simulink model "speedControlSystem"  (R2024b)
settings: Solver=FixedStepAuto  StartTime=0.0  StopTime=Tend  FixedStep=Tsim  RelTol=1e-3
values from neighbouring files (symbols this model uses):
  b = 4.28e-6    (= 4.28e-06)    [setup.m]    (also in test.m)
  encoder_noise_power = 0.5e-6*0    (= 0)    [test.m]
  J = 29.54e-6    (= 2.954e-05)    [test.m]
  speed_ref = 5e3    (= 5000)    [test.m]
  Tend = 10    [computing_speed.m]    (also in setup.m = 0.2; test.m = 0.2)
  Tsim = 1e-5    (= 1e-05)    [computing_speed.m]    (also in setup.m; test.m = 0.0001)
libraries: simulink x1
settings Model: Creator=mhmok  LastModifiedBy=mhmok

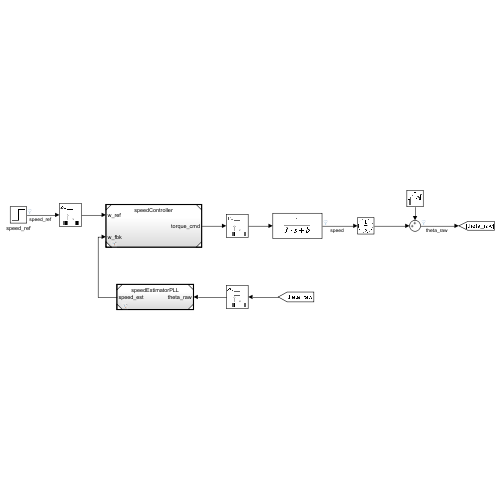
[thumbnail: Simulink's stored preview of the top-level diagram]
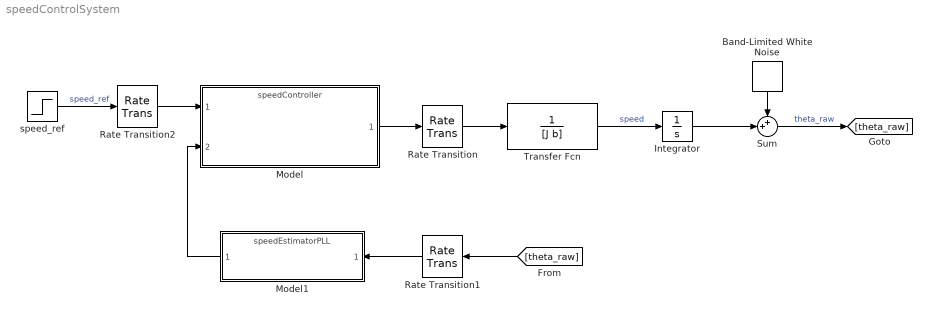
== system speedControlSystem ==
  Band-Limited White Noise : simulink/Sources/Band-Limited White Noise  Cov=[encoder_noise_power]  Ts=Tsim  seed=[23341]
  Integrator : Integrator  WrapState=on  WrappedStateUpperValue=2*pi  WrappedStateLowerValue=0
  Model : ModelReference  ModelNameDialog=speedController.slx  SimulationMode=Normal  ModelReferenceVersion=1.8
  Model1 : ModelReference  ModelNameDialog=speedEstimatorPLL.slx  SimulationMode=Normal  ModelReferenceVersion=1.34
  Rate Transition : RateTransition  OutPortSampleTime=Tsim
  Rate Transition1 : RateTransition  OutPortSampleTime=Ts
  Rate Transition2 : RateTransition  OutPortSampleTime=Ts
  Sum : Sum  Inputs=++|
  Transfer Fcn : TransferFcn  Denominator=[J b]
  speed_ref : Step  Time=Tend/5  After=speed_ref*2*pi/60  SampleTime=0
  wires:
  Rate Transition/1 -> Transfer Fcn/1
  Model/1 -> Rate Transition/1
  Transfer Fcn/1 -> Integrator/1  "speed"
  Rate Transition2/1 -> Model/1
  speed_ref/1 -> Rate Transition2/1  "speed_ref"
  Sum/1 -> [theta_raw]  "theta_raw"
  Band-Limited White Noise/1 -> Sum/1
  Integrator/1 -> Sum/2
  [theta_raw] -> Rate Transition1/1
  Rate Transition1/1 -> Model1/1
  Model1/1 -> Model/2
